simulink model "PI_speed_ctrl"  (Simulink 7.6)
settings: Solver=ode23tb  StartTime=0.0  StopTime=50  FixedStep=1e-3  MaxStep=5e-3  RelTol=1e-3  AbsTol=1e-3
values from neighbouring files (symbols this model uses):
  emTmax = 17e3    (= 17000)    [data_PIspeed.m]
  i = 100, eta=0.95    [data_PIspeed.m]
  Jd_l = 1, Jd_h = 0.5    [data_PIspeed.m]
  Jg = 90    [data_PIspeed.m]
  Jwt = 9e6,    [data_PIspeed.m]
  Lm = 5.09e-3, p = 2    [data_PIspeed.m]
  Ls = 5.25e-3, Lr = 5.25e-3    [data_PIspeed.m]
  ro = 1.25, R= 45    [data_PIspeed.m]
  Rs = 0.004, Rr = 0.004    [data_PIspeed.m]
  sgm = 1-Lm^2/Lr/Ls, Tr=Lr/Rr    [data_PIspeed.m]
  sT = 0    [data_PIspeed.m]
undefined symbols (not defined in the file or in its folder): eta, Jd_h, lam_opt, Lr, p, R, Rr
libraries: simulink x2
settings Model: Creator=Home  LastModifiedBy=Home  ExtModeTrigMode=oneshot  ExtModeArmWhenConnect=off
settings SolverCC: ZeroCrossControl=DisableAll
settings DataIOCC: LimitDataPoints=off  SaveOutput=off  SaveState=on  SaveTime=off  StateSaveName=Pout  SignalLoggingName=sigsOut
settings OptimizationCC: BlockReduction=off  BooleanDataType=off
settings DebuggingCC: SaveWithParameterizedLinksMsg=none  SignalResolutionControl=TryResolveAllWithWarning  SolverPrmCheckMsg=none  MultiTaskDSMMsg=warning  MultiTaskCondExecSysMsg=none  StrictBusMsg=None
settings HardwareCC: TargetUnknown=on
settings RTWCC: IncludeERTFirstTime=on

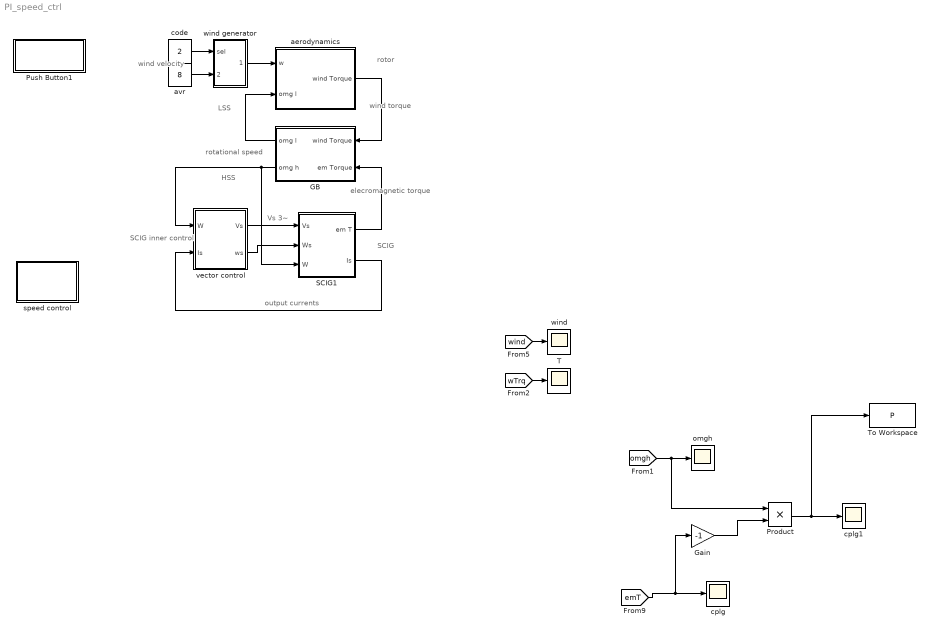
== system PI_speed_ctrl ==
  note: wind
      | torque
  note: LSS
  note: rotational
      | speed
  note: Vs 3~
  note: elecromagnetic
      | torque
  note: SCIG
  note: HSS
  note: SCIG
      | inner
      | control
  note: output currents
  note: rotor
  note: wind
      | velocity
  GB : Subsystem
  Gain : Gain  Gain=-1
  Product : Product  RndMeth=Zero
  Push Button1 : Subsystem
      settings: OpenFcn=data_PIspeed
      mask Display: disp('Double-click to\nload WECS data')
  SCIG1 : Subsystem
  T : Scope
      settings: TimeRange=30  YMin=0  YMax=200  SaveName=cple  DataFormat=Array  MaxDataPoints=2^20
  To Workspace : ToWorkspace  VariableName=P  SampleTime=-1  SaveFormat=Array
  aerodynamics : Subsystem
  avr : Constant  Value=8
  code : Constant  Value=2
  cplg : Scope
      settings: TimeRange=50  YMin=-16000  YMax=2000  SaveName=emT1  DataFormat=Array  MaxDataPoints=2^20
  cplg1 : Scope
      settings: TimeRange=50  YMin=-16000  YMax=2000  SaveName=emT  DataFormat=Array  MaxDataPoints=2^20
  omgh : Scope
      settings: TimeRange=120  YMin=0  YMax=350  SaveName=omgr1  DataFormat=Array  MaxDataPoints=2^20
  speed control : Subsystem
      mask Display: disp('Rotational\nSpeed\nControl')
  vector control : Subsystem
  wind : Scope
      settings: TimeRange=120  YMin=0  YMax=12  SaveName=wind1  DataFormat=Array  MaxDataPoints=2^20
  wind generator : Subsystem
  wires:
  vector control/1(Vs) -> SCIG1/1(Vs)
  SCIG1/1(em T) -> GB/2(em Torque)
  GB/2(omg h) -> SCIG1/3(W), vector control/1(W)
  SCIG1/2(Is) -> vector control/2(Is)
  vector control/2(ws) -> SCIG1/2(Ws)
  aerodynamics/1(" wind Torque") -> GB/1(wind Torque)
  GB/1(omg l) -> aerodynamics/2(omg l)
  code/1 -> wind generator/1(sel)
  avr/1 -> wind generator/2(avr)
  wind generator/1(wind) -> aerodynamics/1(w)
  [omgh] -> omgh/1, Product/1
  [emT] -> cplg/1, Gain/1
  [wTrq] -> T/1
  [wind] -> wind/1
  Gain/1 -> Product/2
  Product/1 -> cplg1/1, To Workspace/1

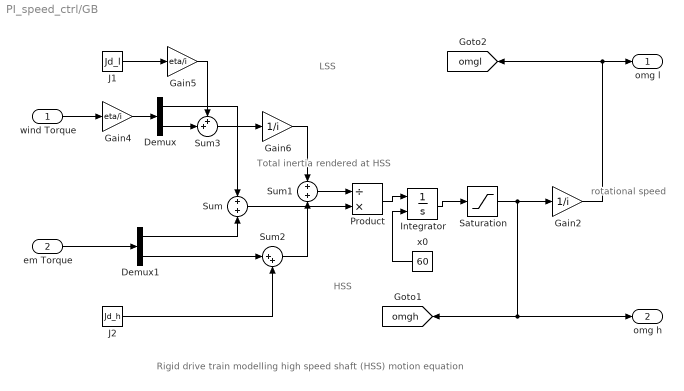
== system PI_speed_ctrl/GB ==
  note: LSS
  note: HSS
  note: Total inertia rendered at HSS
  note: rotational
      | speed
  note: Rigid drive train modelling
      | high speed shaft (HSS) motion equation
  wind Torque : Inport
  em Torque : Inport  Port=2
  Demux : Demux  Outputs=2
  Demux1 : Demux  Outputs=2
  Gain2 : Gain  Gain=1/i  SaturateOnIntegerOverflow=on  OutDataTypeStr=Inherit: Same as input  ParamDataTypeStr=Inherit: Same as input
  Gain4 : Gain  Gain=eta/i  SaturateOnIntegerOverflow=on  OutDataTypeStr=Inherit: Same as input  ParamDataTypeStr=Inherit: Same as input
  Gain5 : Gain  Gain=eta/i  SaturateOnIntegerOverflow=on  OutDataTypeStr=Inherit: Same as input  ParamDataTypeStr=Inherit: Same as input
  Gain6 : Gain  Gain=1/i  SaturateOnIntegerOverflow=on  OutDataTypeStr=Inherit: Same as input  ParamDataTypeStr=Inherit: Same as input
  Integrator : Integrator  InitialConditionSource=external
  J1 : Constant  Value=Jd_l
  J2 : Constant  Value=Jd_h
  Product : Product  Inputs=/*  SaturateOnIntegerOverflow=on  InputSameDT=on  OutDataTypeStr=Inherit: Same as first input
  Saturation : Saturate  UpperLimit=1000  LowerLimit=0
  Sum : Sum  SaturateOnIntegerOverflow=on  InputSameDT=on  OutDataTypeStr=Inherit: Same as first input
  Sum1 : Sum  SaturateOnIntegerOverflow=on  InputSameDT=on  OutDataTypeStr=Inherit: Same as first input
  Sum2 : Sum  Inputs=|++  SaturateOnIntegerOverflow=on  InputSameDT=on  OutDataTypeStr=Inherit: Same as first input
  Sum3 : Sum  Inputs=++|  SaturateOnIntegerOverflow=on  InputSameDT=on  OutDataTypeStr=Inherit: Same as first input
  x0 : Constant  Value=60
  omg l : Outport
  omg h : Outport  Port=2
  tag scope: omgh=global, omgl=global
  wires:
  em Torque/1 -> Demux1/1
  wind Torque/1 -> Gain4/1
  Gain4/1 -> Demux/1
  Demux/1 -> Sum/1
  Demux1/2 -> Sum2/1
  Demux/2 -> Sum3/2
  J2/1 -> Sum2/2
  J1/1 -> Gain5/1
  Gain5/1 -> Sum3/1
  Sum2/1 -> Sum1/2
  Sum3/1 -> Gain6/1
  Gain6/1 -> Sum1/1
  Sum/1 -> Product/2
  Product/1 -> Integrator/1
  Sum1/1 -> Product/1
  Integrator/1 -> Saturation/1
  Saturation/1 -> Gain2/1, omg h/1, [omgh]
  Demux1/1 -> Sum/2
  Gain2/1 -> omg l/1, [omgl]
  x0/1 -> Integrator/2

== system PI_speed_ctrl/Push Button1 ==

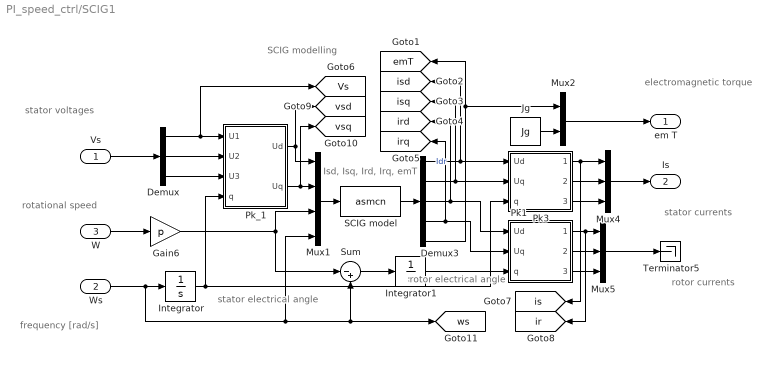
== system PI_speed_ctrl/SCIG1 ==
  note: Isd, Isq,
      | Ird, Irq, emT
  note: SCIG modelling
  note: electromagnetic
      | torque
  note: rotor
      | currents
  note: stator
      | currents
  note: stator
      | voltages
  note: rotational
      | speed
  note: frequency
      | [rad/s]
  note: stator electrical angle
  note: rotor
      | electrical
      | angle
  Vs : Inport
  Ws : Inport  Port=2  SampleTime=0
  W : Inport  Port=3  SampleTime=0
  Demux : Demux  Outputs=3
  Demux3 : Demux  Outputs=5
  Gain6 : Gain  Gain=p  SaturateOnIntegerOverflow=on  OutDataTypeStr=Inherit: Same as input  ParamDataTypeStr=Inherit: Same as input
  Integrator : Integrator
  Integrator1 : Integrator
  Jg : Constant  Value=Jg
  Mux1 : Mux
  Mux2 : Mux  Inputs=2
  Mux4 : Mux  Inputs=3
  Mux5 : Mux  Inputs=3
  Pk1 : Subsystem
      mask Display: disp('2/3')
  Pk3 : Subsystem
      mask Display: disp('2/3')
  Pk_1 : Subsystem
      mask Display: disp('3/2')
  SCIG model : S-Function  FunctionName=asmcn  Parameters=Rs,Rr,Ls,Lr,Lm,p  EnableBusSupport=off
  Sum : Sum  Inputs=|-+  SaturateOnIntegerOverflow=on
  Terminator5 : Terminator
  em T : Outport
  Is : Outport  Port=2
  tag scope: Vs=global, emT=global, ir=global, ird=global, irq=global, is=global, isd=global, isq=global, vsd=global, vsq=global, ws=global
  wires:
  Mux1/1 -> SCIG model/1
  Gain6/1 -> Mux1/3, Sum/1
  Vs/1 -> Demux/1
  Demux/1 -> Pk_1/1(U1), [Vs]
  Demux/2 -> Pk_1/2(U2)
  Demux/3 -> Pk_1/3(U3)
  Ws/1 -> Integrator/1, Mux1/4, Sum/2, [ws]
  W/1 -> Gain6/1
  Integrator/1 -> Pk_1/4(q), Pk3/3(q)
  SCIG model/1 -> Demux3/1
  Demux3/1 -> [isd], Pk3/1(Ud)
  Demux3/2 -> [isq], Pk3/2(Uq)
  Demux3/3 -> Pk1/1(Ud), [ird]  "Idr"
  Demux3/4 -> [irq], Pk1/2(Uq)
  Pk3/1(1) -> Mux4/1, [is]
  Pk1/1(1) -> Mux5/1, [ir]
  Pk3/2(2) -> Mux4/2
  Pk3/3(3) -> Mux4/3
  Pk1/2(2) -> Mux5/2
  Pk1/3(3) -> Mux5/3
  Demux3/5 -> Mux2/1, [emT]
  Jg/1 -> Mux2/2
  Mux2/1 -> em T/1
  Pk_1/1(Ud) -> Mux1/1, [vsd]
  Pk_1/2(Uq) -> Mux1/2, [vsq]
  Mux4/1 -> Is/1
  Mux5/1 -> Terminator5/1
  Sum/1 -> Integrator1/1
  Integrator1/1 -> Pk1/3(q)

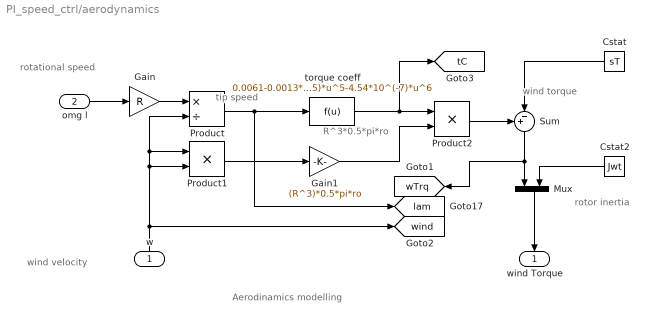
== system PI_speed_ctrl/aerodynamics ==
  note: wind
      | torque
  note: R^3*0.5*pi*ro
  note: Aerodinamics modelling
  note: wind
      | velocity
  note: rotational
      | speed
  note: rotor
      | inertia
  note: tip speed
  w : Inport
  omg l : Inport  Port=2
  Cstat : Constant  Value=sT
  Cstat2 : Constant  Value=Jwt
  Gain : Gain  Gain=R  SaturateOnIntegerOverflow=on  OutDataTypeStr=Inherit: Same as input  ParamDataTypeStr=Inherit: Same as input
  Gain1 : Gain  Gain=(R^3)*0.5*pi*ro  SaturateOnIntegerOverflow=on  OutDataTypeStr=Inherit: Same as input  ParamDataTypeStr=Inherit: Same as input
  Mux : Mux  Inputs=2
  Product : Product  Inputs=*/  SaturateOnIntegerOverflow=on  InputSameDT=on  OutDataTypeStr=Inherit: Same as first input
  Product1 : Product  SaturateOnIntegerOverflow=on  InputSameDT=on  OutDataTypeStr=Inherit: Same as first input
  Product2 : Product  SaturateOnIntegerOverflow=on  InputSameDT=on  OutDataTypeStr=Inherit: Same as first input
  Sum : Sum  Inputs=+-|  SaturateOnIntegerOverflow=on  InputSameDT=on  OutDataTypeStr=Inherit: Same as first input
  "torque coeff " : Fcn  Expr=0.0061-0.0013*u+0.0081*u^2-9.7477*10^(-4)*u^3-6.5416*10^(-5)*u^4+1.3027*10^(-5)*u^5-4.54*10^(-7)*u^6
  " wind Torque" : Outport
  tag scope: lam=global, tC=global, wTrq=global, wind=global
  wires:
  Product/1 -> "torque coeff "/1, [lam]
  Gain/1 -> Product/1
  Product1/1 -> Gain1/1
  Gain1/1 -> Product2/2
  "torque coeff "/1 -> Product2/1, [tC]
  Product2/1 -> Sum/1
  omg l/1 -> Gain/1
  w/1 -> Product/2, Product1/1, Product1/2, [wind]
  Mux/1 -> " wind Torque"/1
  Cstat2/1 -> Mux/2
  Sum/1 -> [wTrq], Mux/1
  Cstat/1 -> Sum/2

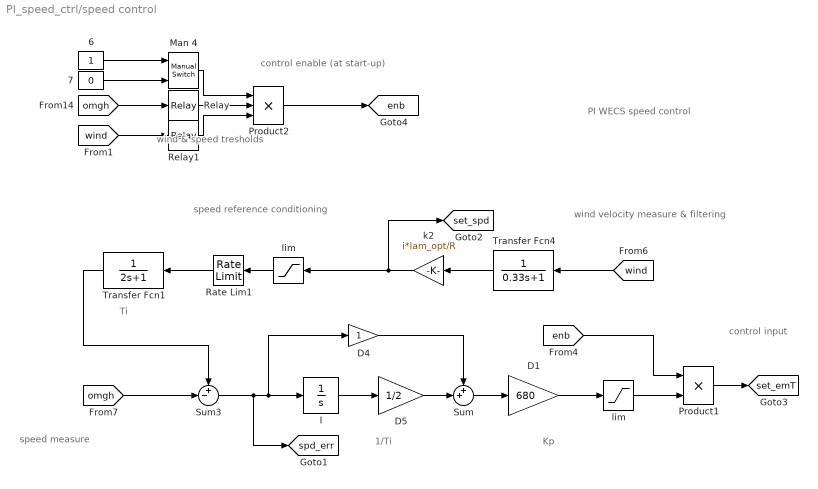
== system PI_speed_ctrl/speed control ==
  note: 1/Ti
  note: speed measure
  note: control input
  note: control enable
      | (at start-up)
  note: wind velocity
      | measure & filtering
  note: speed reference conditioning
  note: Kp
  note: PI WECS
      | speed control
  note: wind & speed tresholds
  note: Ti
  " lim" : Saturate  UpperLimit=emTmax/15  LowerLimit=-emTmax
  6 : Constant
  7 : Constant  Value=0
  D1 : Gain  Gain=680  SaturateOnIntegerOverflow=on  OutDataTypeStr=Inherit: Same as input  ParamDataTypeStr=Inherit: Same as input
  D4 : Gain  SaturateOnIntegerOverflow=on  OutDataTypeStr=Inherit: Same as input  ParamDataTypeStr=Inherit: Same as input
  D5 : Gain  Gain=1/2  SaturateOnIntegerOverflow=on  OutDataTypeStr=Inherit: Same as input  ParamDataTypeStr=Inherit: Same as input
  I : TransferFcn  Denominator=[1 0]
  Man 4 : simulink/Signal Routing/Manual Switch  SystemSampleTime=-1  sw=1  action=0  varsize=off
  Product1 : Product  SaturateOnIntegerOverflow=on  InputSameDT=on  OutDataTypeStr=Inherit: Same as first input
  Product2 : Product  Inputs=3  SaturateOnIntegerOverflow=on  InputSameDT=on  OutDataTypeStr=Inherit: Same as first input
  Rate Lim1 : RateLimiter  RisingSlewLimit=1000  FallingSlewLimit=-1000
  Relay : Relay  OnSwitchValue=100  OffSwitchValue=0
  Relay1 : Relay  OnSwitchValue=4  OffSwitchValue=0
  Sum : Sum  Inputs=++|  SaturateOnIntegerOverflow=on  InputSameDT=on  OutDataTypeStr=Inherit: Same as first input
  Sum3 : Sum  Inputs=+-|  SaturateOnIntegerOverflow=on  InputSameDT=on  OutDataTypeStr=Inherit: Same as first input
  Transfer Fcn1 : TransferFcn  Denominator=[2 1]
  Transfer Fcn4 : TransferFcn  Denominator=[0.33 1]
  k2 : Gain  Gain=i*lam_opt/R  SaturateOnIntegerOverflow=on  OutDataTypeStr=Inherit: Same as input  ParamDataTypeStr=Inherit: Same as input
  lim : Saturate  UpperLimit=300  LowerLimit=0
  tag scope: enb=global, set_emT=global, set_spd=global, spd_err=global
  wires:
  [wind] -> Transfer Fcn4/1
  Transfer Fcn4/1 -> k2/1
  lim/1 -> Rate Lim1/1
  Rate Lim1/1 -> Transfer Fcn1/1
  Product2/1 -> [enb]
  Man 4/1 -> Product2/1
  7/1 -> Man 4/2
  6/1 -> Man 4/1
  Relay/1 -> Product2/2
  [wind] -> Relay1/1
  [omgh] -> Relay/1
  Relay1/1 -> Product2/3
  k2/1 -> lim/1, [set_spd]
  Sum/1 -> D1/1
  I/1 -> D5/1
  Sum3/1 -> D4/1, I/1, [spd_err]
  D1/1 -> " lim"/1
  D4/1 -> Sum/1
  D5/1 -> Sum/2
  [omgh] -> Sum3/2
  [enb] -> Product1/1
  " lim"/1 -> Product1/2
  Product1/1 -> [set_emT]
  Transfer Fcn1/1 -> Sum3/1

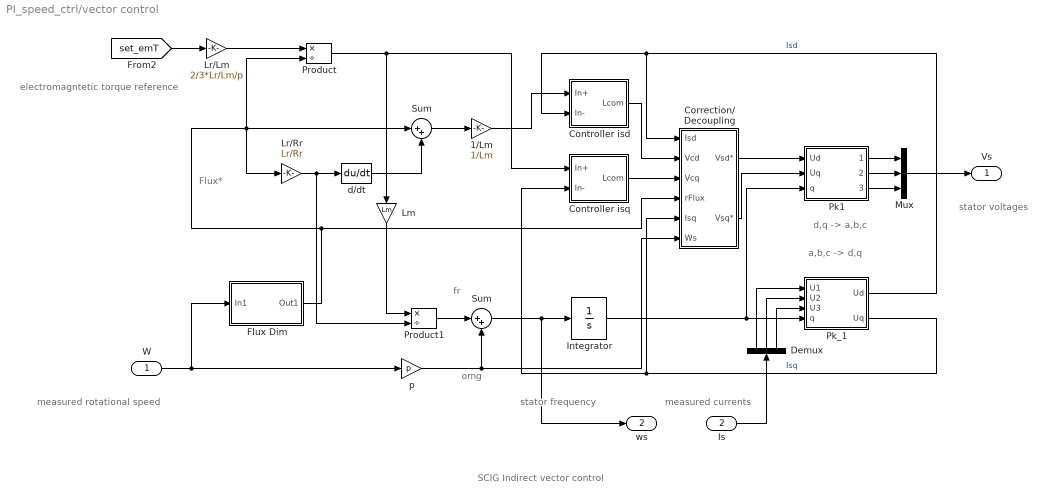
== system PI_speed_ctrl/vector control ==
  note: a,b,c -> d,q
  note: stator frequency
  note: measured currents
  note: stator
      | voltages
  note: d,q -> a,b,c
  note: measured
      | rotational speed
  note: electromagntetic
      | torque reference
  note: SCIG Indirect vector control
  note: fr
  note: omg
  note: Flux*
  W : Inport
  Is : Inport  Port=2
  1/Lm : Gain  Gain=1/Lm  SaturateOnIntegerOverflow=on  OutDataTypeStr=Inherit: Same as input  ParamDataTypeStr=Inherit: Same as input
  Controller isd : Subsystem  TreatAsAtomicUnit=on  mask(PI){Kp=0.8, Ki=1000, lim=1000, awu=1}
      mask prompts: Kp "Proportional:"; Ki "Integral:"; lim "Limit:"; awu "Anti W-up (y/n)?"
      mask Display:
      | disp('+In          \n\n')
      | disp('PI')
      | disp('\n\n-In         ')
  Controller isq : Subsystem  TreatAsAtomicUnit=on  mask(PI){Kp=0.8, Ki=800, lim=1000, awu=1}
      mask prompts: Kp "Proportional:"; Ki "Integral:"; lim "Limit:"; awu "Anti W-up (y/n)?"
      mask Display:
      | disp('+In          \n\n')
      | disp('PI')
      | disp('\n\n-In         ')
  Correction/ Decoupling : Subsystem  TreatAsAtomicUnit=on
  Demux : Demux  Outputs=3
  Flux Dim : Subsystem  mask{frref=0.88, omgn=200, cd=2}
      mask prompts: frref "Set point flux [Wb]:"; omgn "Wn [rad/s]:"; cd "Coef. dim. flux :"
      mask init:
      | x=-1:0.1:0;
      mask Display:
      | plot(-1.2,1.5,1.7,0.95)
      | plot([-1,0.5],[1.415,1.415]),
      | plot([-0.75,-0.75],[0.98,1.48],[-1,1.55],[1,1])
      | plot( x+1.5,sqrt(1+x.^2)),
  Integrator : Integrator
  Lm : Gain  Gain=Lm  SaturateOnIntegerOverflow=on  OutDataTypeStr=Inherit: Same as input  ParamDataTypeStr=Inherit: Same as input
  Lr/Lm : Gain  Gain=2/3*Lr/Lm/p  SaturateOnIntegerOverflow=on  OutDataTypeStr=Inherit: Same as input  ParamDataTypeStr=Inherit: Same as input
  Lr/Rr : Gain  Gain=Lr/Rr  SaturateOnIntegerOverflow=on  OutDataTypeStr=Inherit: Same as input  ParamDataTypeStr=Inherit: Same as input
  Mux : Mux  Inputs=3
  Pk1 : Subsystem
      mask Display: disp('2/3')
  Pk_1 : Subsystem
      mask Display: disp('3/2')
  Product : Product  Inputs=*/  SaturateOnIntegerOverflow=on  InputSameDT=on  OutDataTypeStr=Inherit: Same as first input
  Product1 : Product  Inputs=*/  SaturateOnIntegerOverflow=on  InputSameDT=on  OutDataTypeStr=Inherit: Same as first input
  Sum : Sum  Inputs=|++  SaturateOnIntegerOverflow=on  InputSameDT=on  OutDataTypeStr=Inherit: Same as first input
  "Sum " : Sum  Inputs=|++  SaturateOnIntegerOverflow=on  InputSameDT=on  OutDataTypeStr=Inherit: Same as first input
  d/dt : Derivative
  p : Gain  Gain=p  SaturateOnIntegerOverflow=on  OutDataTypeStr=Inherit: Same as input  ParamDataTypeStr=Inherit: Same as input
  Vs : Outport
  ws : Outport  Port=2
  wires:
  Flux Dim/1(Out1) -> Product/2, "Sum "/1, Lr/Rr/1, Correction/ Decoupling/4(rFlux)
  Integrator/1 -> Pk_1/4(q), Pk1/3(q)
  W/1 -> Flux Dim/1(In1), p/1
  Controller isq/1(Lcom) -> Correction/ Decoupling/3(Vcq)
  Pk_1/2(Uq) -> Controller isq/2(In-), Correction/ Decoupling/5(Isq)  "Isq"
  Pk1/1(1) -> Mux/1
  Pk1/2(2) -> Mux/2
  Pk1/3(3) -> Mux/3
  Mux/1 -> Vs/1
  Pk_1/1(Ud) -> Correction/ Decoupling/1(Isd), Controller isd/2(In-)  "Isd"
  Controller isd/1(Lcom) -> Correction/ Decoupling/2(Vcd)
  Correction/ Decoupling/2(Vsq*) -> Pk1/2(Uq)
  Correction/ Decoupling/1(Vsd*) -> Pk1/1(Ud)
  Sum/1 -> ws/1, Integrator/1
  "Sum "/1 -> 1/Lm/1
  Lm/1 -> Product1/1
  Is/1 -> Demux/1
  Demux/1 -> Pk_1/1(U1)
  Demux/2 -> Pk_1/2(U2)
  Demux/3 -> Pk_1/3(U3)
  [set_emT] -> Lr/Lm/1
  Lr/Rr/1 -> d/dt/1, Product1/2
  Lr/Lm/1 -> Product/1
  Product/1 -> Controller isq/1(In+), Lm/1
  Product1/1 -> Sum/1
  d/dt/1 -> "Sum "/2
  1/Lm/1 -> Controller isd/1(In+)
  p/1 -> Sum/2, Correction/ Decoupling/6(Ws)

== system PI_speed_ctrl/wind generator ==
  note: wind velocity sequence
      | generator & selector
  note: 1
  note: 2
  note: 3
  note: 4
  note: 5
  note: constant
  note: selection
  note: average
  sel : Inport
  avr : Inport  Port=2
  Switch : MultiPortSwitch  Inputs=5  zeroidx=off  SaturateOnIntegerOverflow=on
  filter shape1 : Subsystem
  filter shape2 : Subsystem
  filter shape3 : Subsystem
  pre-computed : Subsystem
  wind : Outport
  wires:
  avr/1 -> Switch/2, filter shape1/1(avr), filter shape2/1(avr), filter shape3/1(avr), pre-computed/1(avr)
  sel/1 -> Switch/1
  Switch/1 -> wind/1
  filter shape1/1(w) -> Switch/3
  pre-computed/1(w) -> Switch/5
  filter shape3/1(w) -> Switch/6
  filter shape2/1(w) -> Switch/4

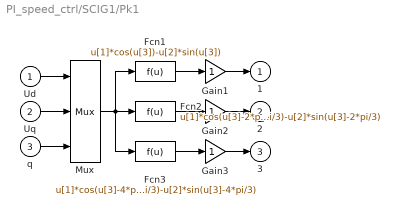
== system PI_speed_ctrl/SCIG1/Pk1 ==
  Ud : Inport
  Uq : Inport  Port=2
  q : Inport  Port=3
  Fcn1 : Fcn  Expr=u[1]*cos(u[3])-u[2]*sin(u[3])
  Fcn2 : Fcn  Expr=u[1]*cos(u[3]-2*pi/3)-u[2]*sin(u[3]-2*pi/3)
  Fcn3 : Fcn  Expr=u[1]*cos(u[3]-4*pi/3)-u[2]*sin(u[3]-4*pi/3)
  Gain1 : Gain  SaturateOnIntegerOverflow=on  OutDataTypeStr=Inherit: Same as input  ParamDataTypeStr=Inherit: Same as input
  Gain2 : Gain  SaturateOnIntegerOverflow=on  OutDataTypeStr=Inherit: Same as input  ParamDataTypeStr=Inherit: Same as input
  Gain3 : Gain  SaturateOnIntegerOverflow=on  OutDataTypeStr=Inherit: Same as input  ParamDataTypeStr=Inherit: Same as input
  Mux : Mux  Inputs=3
  1 : Outport
  2 : Outport  Port=2
  3 : Outport  Port=3
  wires:
  q/1 -> Mux/3
  Uq/1 -> Mux/2
  Ud/1 -> Mux/1
  Mux/1 -> Fcn2/1, Fcn3/1, Fcn1/1
  Fcn1/1 -> Gain1/1
  Fcn2/1 -> Gain2/1
  Fcn3/1 -> Gain3/1
  Gain3/1 -> 3/1
  Gain2/1 -> 2/1
  Gain1/1 -> 1/1

== system PI_speed_ctrl/SCIG1/Pk3 ==
  note: Park inv
  Ud : Inport
  Uq : Inport  Port=2
  q : Inport  Port=3
  Fcn1 : Fcn  Expr=u[1]*cos(u[3])-u[2]*sin(u[3])
  Fcn2 : Fcn  Expr=u[1]*cos(u[3]-2*pi/3)-u[2]*sin(u[3]-2*pi/3)
  Fcn3 : Fcn  Expr=u[1]*cos(u[3]-4*pi/3)-u[2]*sin(u[3]-4*pi/3)
  Mux : Mux  Inputs=3
  1 : Outport
  2 : Outport  Port=2
  3 : Outport  Port=3
  wires:
  Fcn3/1 -> 3/1
  Fcn2/1 -> 2/1
  Fcn1/1 -> 1/1
  Mux/1 -> Fcn1/1, Fcn3/1, Fcn2/1
  Ud/1 -> Mux/1
  Uq/1 -> Mux/2
  q/1 -> Mux/3

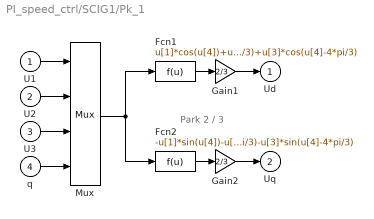
== system PI_speed_ctrl/SCIG1/Pk_1 ==
  note: Park 2 / 3
  U1 : Inport
  U2 : Inport  Port=2
  U3 : Inport  Port=3
  q : Inport  Port=4
  Fcn1 : Fcn  Expr=u[1]*cos(u[4])+u[2]*cos(u[4]-2*pi/3)+u[3]*cos(u[4]-4*pi/3)
  Fcn2 : Fcn  Expr=-u[1]*sin(u[4])-u[2]*sin(u[4]-2*pi/3)-u[3]*sin(u[4]-4*pi/3)
  Gain1 : Gain  Gain=2/3  SaturateOnIntegerOverflow=on  OutDataTypeStr=Inherit: Same as input  ParamDataTypeStr=Inherit: Same as input
  Gain2 : Gain  Gain=2/3  SaturateOnIntegerOverflow=on  OutDataTypeStr=Inherit: Same as input  ParamDataTypeStr=Inherit: Same as input
  Mux : Mux
  Ud : Outport
  Uq : Outport  Port=2
  wires:
  Gain2/1 -> Uq/1
  Fcn2/1 -> Gain2/1
  Fcn1/1 -> Gain1/1
  Gain1/1 -> Ud/1
  Mux/1 -> Fcn1/1, Fcn2/1
  q/1 -> Mux/4
  U3/1 -> Mux/3
  U2/1 -> Mux/2
  U1/1 -> Mux/1

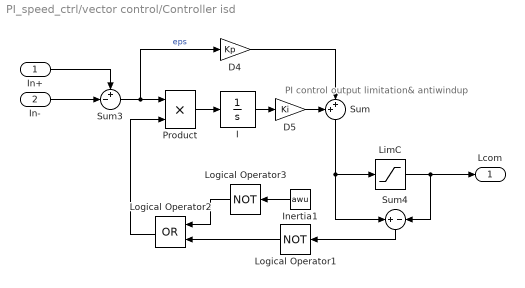
== system PI_speed_ctrl/vector control/Controller isd ==
  note: PI control
      | output limitation& antiwindup
  In+ : Inport
  In- : Inport  Port=2
  D4 : Gain  Gain=Kp  SaturateOnIntegerOverflow=on  OutDataTypeStr=Inherit: Same as input  ParamDataTypeStr=Inherit: Same as input
  D5 : Gain  Gain=Ki  SaturateOnIntegerOverflow=on  OutDataTypeStr=Inherit: Same as input  ParamDataTypeStr=Inherit: Same as input
  I : TransferFcn  Denominator=[1 0]
  Inertia1 : Constant  Value=awu
  LimC : Saturate  UpperLimit=lim  LowerLimit=-lim
  Logical Operator1 : Logic  Operator=NOT
  Logical Operator2 : Logic  Operator=OR
  Logical Operator3 : Logic  Operator=NOT
  Product : Product  SaturateOnIntegerOverflow=on  InputSameDT=on  OutDataTypeStr=Inherit: Same as first input
  Sum : Sum  Inputs=++|  SaturateOnIntegerOverflow=on  InputSameDT=on  OutDataTypeStr=Inherit: Same as first input
  Sum3 : Sum  Inputs=+-|  SaturateOnIntegerOverflow=on  InputSameDT=on  OutDataTypeStr=Inherit: Same as first input
  Sum4 : Sum  Inputs=+|-  SaturateOnIntegerOverflow=on  InputSameDT=on  OutDataTypeStr=Inherit: Same as first input
  Lcom : Outport
  wires:
  Sum3/1 -> Product/1, D4/1  "eps"
  Product/1 -> I/1
  In-/1 -> Sum3/2
  In+/1 -> Sum3/1
  I/1 -> D5/1
  D5/1 -> Sum/1
  D4/1 -> Sum/2
  LimC/1 -> Sum4/2, Lcom/1
  Sum/1 -> LimC/1, Sum4/1
  Logical Operator1/1 -> Logical Operator2/2
  Inertia1/1 -> Logical Operator3/1
  Logical Operator3/1 -> Logical Operator2/1
  Logical Operator2/1 -> Product/2
  Sum4/1 -> Logical Operator1/1

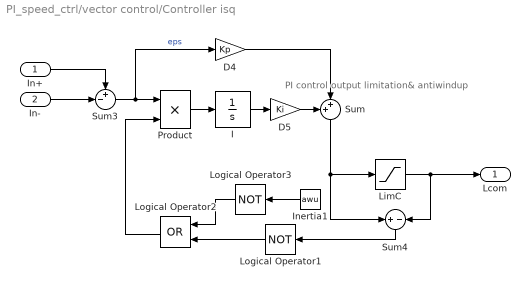
== system PI_speed_ctrl/vector control/Controller isq ==
  note: PI control
      | output limitation& antiwindup
  In+ : Inport
  In- : Inport  Port=2
  D4 : Gain  Gain=Kp  SaturateOnIntegerOverflow=on  OutDataTypeStr=Inherit: Same as input  ParamDataTypeStr=Inherit: Same as input
  D5 : Gain  Gain=Ki  SaturateOnIntegerOverflow=on  OutDataTypeStr=Inherit: Same as input  ParamDataTypeStr=Inherit: Same as input
  I : TransferFcn  Denominator=[1 0]
  Inertia1 : Constant  Value=awu
  LimC : Saturate  UpperLimit=lim  LowerLimit=-lim
  Logical Operator1 : Logic  Operator=NOT
  Logical Operator2 : Logic  Operator=OR
  Logical Operator3 : Logic  Operator=NOT
  Product : Product  SaturateOnIntegerOverflow=on  InputSameDT=on  OutDataTypeStr=Inherit: Same as first input
  Sum : Sum  Inputs=++|  SaturateOnIntegerOverflow=on  InputSameDT=on  OutDataTypeStr=Inherit: Same as first input
  Sum3 : Sum  Inputs=+-|  SaturateOnIntegerOverflow=on  InputSameDT=on  OutDataTypeStr=Inherit: Same as first input
  Sum4 : Sum  Inputs=+|-  SaturateOnIntegerOverflow=on  InputSameDT=on  OutDataTypeStr=Inherit: Same as first input
  Lcom : Outport
  wires:
  Sum4/1 -> Logical Operator1/1
  Logical Operator2/1 -> Product/2
  Logical Operator3/1 -> Logical Operator2/1
  Inertia1/1 -> Logical Operator3/1
  Logical Operator1/1 -> Logical Operator2/2
  Sum/1 -> Sum4/1, LimC/1
  LimC/1 -> Lcom/1, Sum4/2
  D4/1 -> Sum/2
  D5/1 -> Sum/1
  I/1 -> D5/1
  In+/1 -> Sum3/1
  In-/1 -> Sum3/2
  Product/1 -> I/1
  Sum3/1 -> D4/1, Product/1  "eps"

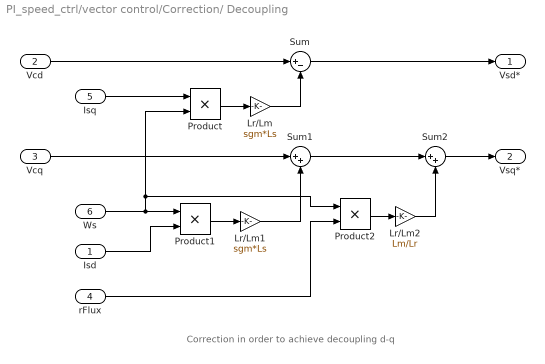
== system PI_speed_ctrl/vector control/Correction/ Decoupling ==
  note: Correction in order to achieve decoupling d-q
  Isd : Inport
  Vcd : Inport  Port=2
  Vcq : Inport  Port=3
  rFlux : Inport  Port=4
  Isq : Inport  Port=5
  Ws : Inport  Port=6
  Lr/Lm : Gain  Gain=sgm*Ls  SaturateOnIntegerOverflow=on  OutDataTypeStr=Inherit: Same as input  ParamDataTypeStr=Inherit: Same as input
  Lr/Lm1 : Gain  Gain=sgm*Ls  SaturateOnIntegerOverflow=on  OutDataTypeStr=Inherit: Same as input  ParamDataTypeStr=Inherit: Same as input
  Lr/Lm2 : Gain  Gain=Lm/Lr  SaturateOnIntegerOverflow=on  OutDataTypeStr=Inherit: Same as input  ParamDataTypeStr=Inherit: Same as input
  Product : Product  SaturateOnIntegerOverflow=on  InputSameDT=on  OutDataTypeStr=Inherit: Same as first input
  Product1 : Product  SaturateOnIntegerOverflow=on  InputSameDT=on  OutDataTypeStr=Inherit: Same as first input
  Product2 : Product  SaturateOnIntegerOverflow=on  InputSameDT=on  OutDataTypeStr=Inherit: Same as first input
  Sum : Sum  Inputs=|+-  SaturateOnIntegerOverflow=on  InputSameDT=on  OutDataTypeStr=Inherit: Same as first input
  Sum1 : Sum  Inputs=|++  SaturateOnIntegerOverflow=on  InputSameDT=on  OutDataTypeStr=Inherit: Same as first input
  Sum2 : Sum  Inputs=|++  SaturateOnIntegerOverflow=on  InputSameDT=on  OutDataTypeStr=Inherit: Same as first input
  Vsd* : Outport
  Vsq* : Outport  Port=2
  wires:
  Lr/Lm/1 -> Sum/2
  Product/1 -> Lr/Lm/1
  Isq/1 -> Product/1
  Lr/Lm1/1 -> Sum1/2
  Product1/1 -> Lr/Lm1/1
  Lr/Lm2/1 -> Sum2/2
  Ws/1 -> Product1/1, Product2/1, Product/2
  Product2/1 -> Lr/Lm2/1
  rFlux/1 -> Product2/2
  Isd/1 -> Product1/2
  Sum1/1 -> Sum2/1
  Sum2/1 -> Vsq*/1
  Vcd/1 -> Sum/1
  Sum/1 -> Vsd*/1
  Vcq/1 -> Sum1/1

== system PI_speed_ctrl/vector control/Flux Dim ==
  In1 : Inport
  Fcn1 : Fcn  Expr=frref/(1+u[1]*(u[2]-omgn)/(omgn/cd))
  Mux : Mux  Inputs=2
  Relay1 : Relay  OnSwitchValue=omgn  OffSwitchValue=omgn
  Out1 : Outport
  wires:
  Mux/1 -> Fcn1/1
  Relay1/1 -> Mux/1
  In1/1 -> Mux/2, Relay1/1
  Fcn1/1 -> Out1/1

== system PI_speed_ctrl/vector control/Pk1 ==
  note: Park inv
  Ud : Inport
  Uq : Inport  Port=2
  q : Inport  Port=3
  Fcn1 : Fcn  Expr=u[1]*cos(u[3])-u[2]*sin(u[3])
  Fcn2 : Fcn  Expr=u[1]*cos(u[3]-2*pi/3)-u[2]*sin(u[3]-2*pi/3)
  Fcn3 : Fcn  Expr=u[1]*cos(u[3]-4*pi/3)-u[2]*sin(u[3]-4*pi/3)
  Mux : Mux  Inputs=3
  1 : Outport
  2 : Outport  Port=2
  3 : Outport  Port=3
  wires:
  Fcn3/1 -> 3/1
  Fcn2/1 -> 2/1
  Fcn1/1 -> 1/1
  Mux/1 -> Fcn1/1, Fcn3/1, Fcn2/1
  Ud/1 -> Mux/1
  Uq/1 -> Mux/2
  q/1 -> Mux/3

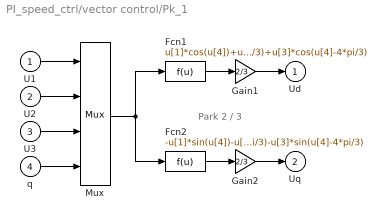
== system PI_speed_ctrl/vector control/Pk_1 ==
  note: Park 2 / 3
  U1 : Inport
  U2 : Inport  Port=2
  U3 : Inport  Port=3
  q : Inport  Port=4
  Fcn1 : Fcn  Expr=u[1]*cos(u[4])+u[2]*cos(u[4]-2*pi/3)+u[3]*cos(u[4]-4*pi/3)
  Fcn2 : Fcn  Expr=-u[1]*sin(u[4])-u[2]*sin(u[4]-2*pi/3)-u[3]*sin(u[4]-4*pi/3)
  Gain1 : Gain  Gain=2/3  SaturateOnIntegerOverflow=on  OutDataTypeStr=Inherit: Same as input  ParamDataTypeStr=Inherit: Same as input
  Gain2 : Gain  Gain=2/3  SaturateOnIntegerOverflow=on  OutDataTypeStr=Inherit: Same as input  ParamDataTypeStr=Inherit: Same as input
  Mux : Mux
  Ud : Outport
  Uq : Outport  Port=2
  wires:
  U1/1 -> Mux/1
  U2/1 -> Mux/2
  U3/1 -> Mux/3
  q/1 -> Mux/4
  Mux/1 -> Fcn2/1, Fcn1/1
  Gain1/1 -> Ud/1
  Fcn1/1 -> Gain1/1
  Fcn2/1 -> Gain2/1
  Gain2/1 -> Uq/1

== system PI_speed_ctrl/wind generator/filter shape1 ==
  avr : Inport
  Random Number : RandomNumber  SampleTime=1e-1
  Random Number1 : RandomNumber  Seed=10000  SampleTime=1e-1
  Sum2 : Sum  Inputs=+++  SaturateOnIntegerOverflow=on  InputSameDT=on  OutDataTypeStr=Inherit: Same as first input
  Transfer Fcn1 : TransferFcn  Denominator=[0.5 1]
  Transfer Fcn2 : TransferFcn  Numerator=[20]  Denominator=[20 1]
  Transfer Fcn3 : TransferFcn  Numerator=[4]  Denominator=[0.5 1]
  Transfer Fcn4 : TransferFcn  Denominator=[20 1]
  w : Outport
  wires:
  Sum2/1 -> w/1
  Transfer Fcn1/1 -> Sum2/2
  Transfer Fcn3/1 -> Transfer Fcn1/1
  Random Number1/1 -> Transfer Fcn3/1
  Transfer Fcn4/1 -> Sum2/1
  avr/1 -> Sum2/3
  Random Number/1 -> Transfer Fcn2/1
  Transfer Fcn2/1 -> Transfer Fcn4/1

== system PI_speed_ctrl/wind generator/filter shape2 ==
  avr : Inport
  Band-Limited White Noise : simulink/Sources/Band-Limited White Noise  SystemSampleTime=-1  Cov=[0.1]  Ts=0.1  seed=[23341]
  Sum : Sum  Inputs=+++  SaturateOnIntegerOverflow=on
  Transfer Fcn : TransferFcn  Numerator=[4]  Denominator=[10 1]
  Transfer Fcn1 : TransferFcn  Numerator=[20]  Denominator=[50 1]
  w : Outport
  wires:
  Band-Limited White Noise/1 -> Transfer Fcn1/1, Transfer Fcn/1
  Transfer Fcn/1 -> Sum/1
  Transfer Fcn1/1 -> Sum/2
  Sum/1 -> w/1
  avr/1 -> Sum/3

== system PI_speed_ctrl/wind generator/filter shape3 ==
  avr : Inport
  Random Number : RandomNumber  SampleTime=1e-1
  Random Number1 : RandomNumber  Seed=10000  SampleTime=1e-1
  Sum2 : Sum  Inputs=+++  SaturateOnIntegerOverflow=on  InputSameDT=on  OutDataTypeStr=Inherit: Same as first input
  Transfer Fcn : TransferFcn  Numerator=[2]  Denominator=[4 1]
  Transfer Fcn1 : TransferFcn  Numerator=[35]  Denominator=[40 1]
  w : Outport
  wires:
  Transfer Fcn/1 -> Sum2/1
  Random Number/1 -> Transfer Fcn/1
  avr/1 -> Sum2/3
  Random Number1/1 -> Transfer Fcn1/1
  Transfer Fcn1/1 -> Sum2/2
  Sum2/1 -> w/1

== system PI_speed_ctrl/wind generator/pre-computed ==
  avr : Inport
  "- avr " : Constant  Value=-7
  Sum1 : Sum  SaturateOnIntegerOverflow=on  InputSameDT=on  OutDataTypeStr=Inherit: Same as first input
  Sum2 : Sum  SaturateOnIntegerOverflow=on  InputSameDT=on  OutDataTypeStr=Inherit: Same as first input
  Transfer Fcn4 : TransferFcn  Denominator=[0.2 1]
  pre-computed wind : FromWorkspace  VariableName=[tt vK]  SampleTime=0.1
  w : Outport
  wires:
  pre-computed wind/1 -> Sum2/1
  "- avr "/1 -> Sum2/2
  Sum2/1 -> Transfer Fcn4/1
  avr/1 -> Sum1/1
  Transfer Fcn4/1 -> Sum1/2
  Sum1/1 -> w/1
